simulink model "rigLoggerRigH"  (R2012b)
settings: Solver=FixedStepDiscrete  StartTime=0.0  StopTime=10.0  FixedStep=0.001  RelTol=1e-3
undefined symbols (not defined in the file or in its folder): macaddr
libraries: Lib_FileLogger x10, xpcnetworkbufferlib x1, xpcethernetlib x1
settings Model: BufferReuse=off  Creator=gilja  LastModifiedBy=Chethan
settings SolverCC: EnableConcurrentExecution=on  ConcurrentTasks=on
settings DataIOCC: SaveOutput=off  SignalLogging=off  SaveTime=off
settings OptimizationCC: InlineParams=on  InlineInvariantSignals=on  OptimizeBlockIOStorage=off  BufferReuse=off  ExpressionFolding=off  LocalBlockOutputs=off  SimCompilerOptimization=On
settings HardwareCC: ProdIntDivRoundTo=Zero  ProdEndianess=LittleEndian  ProdHWDeviceType=Generic->32-bit x86 compatible
settings ModelReferenceCC: ModelReferenceNumInstancesAllowed=Single  ModelReferenceMinAlgLoopOccurrences=on
settings RTWCC: SystemTargetFile=xpctarget.tlc  TemplateMakefile=xpc_default_tmf  Description=xPC Target  ProcessScript=xpctarget_make_rtw_hook  RTWCompilerOptimization=On
settings CodeAppCC: MaxIdLength=62
settings xpcTargetCC: TargetFcnLib=ansi_tfl_table_tmw.mat  CodeReplacementLibrary=XPC_BLAS  ParMdlRefBuildCompliant=on  ConcurrentExecutionCompliant=on  CombineSignalStateStructs=off  GRTInterface=on  RL32LogTETModifier=off  xPCTaskExecutionProfile=off  xPCRL32EventNumber=5000  xPCisDownloadable=off  xPCLoadParamSetFile=off  xPCConcurrentTasks=off  xPCEnableSFAnimation=off

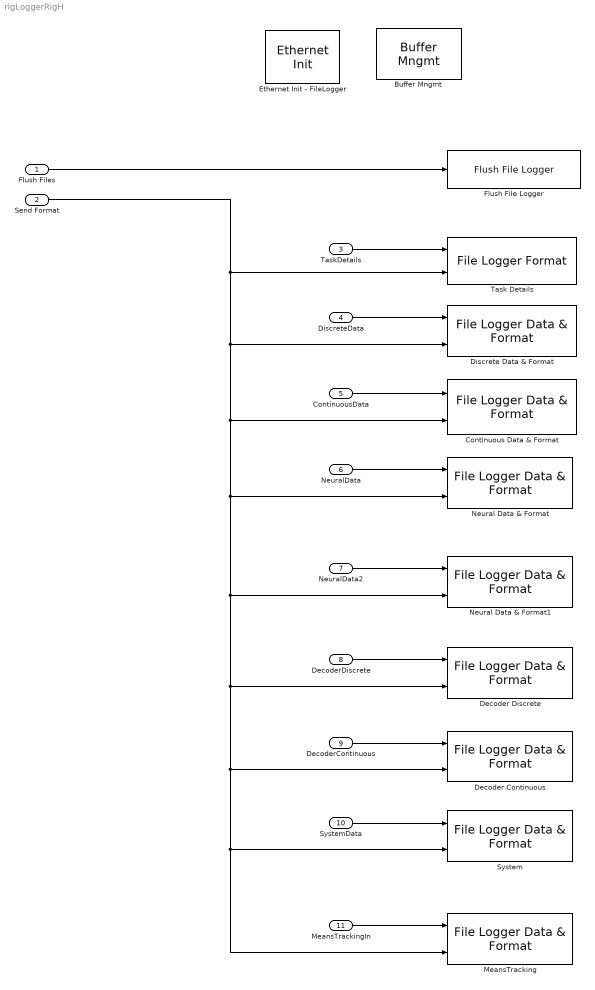
== system rigLoggerRigH ==
  Flush Files : Inport  OutDataTypeStr=boolean
  Send Format : Inport  Port=2  OutDataTypeStr=boolean
  TaskDetails : Inport  Port=3  OutDataTypeStr=Bus: fileLoggerFormat
  DiscreteData : Inport  Port=4  OutDataTypeStr=Bus: fileLoggerFormatAndData
  ContinuousData : Inport  Port=5  OutDataTypeStr=Bus: fileLoggerFormatAndData
  NeuralData : Inport  Port=6  OutDataTypeStr=Bus: fileLoggerFormatAndData
  NeuralData2 : Inport  Port=7  OutDataTypeStr=Bus: fileLoggerFormatAndData
  DecoderDiscrete : Inport  Port=8  OutDataTypeStr=Bus: fileLoggerFormatAndData
  DecoderContinuous : Inport  Port=9  OutDataTypeStr=Bus: fileLoggerFormatAndData
  SystemData : Inport  Port=10  OutDataTypeStr=Bus: fileLoggerFormatAndData
  MeansTrackingIn : Inport  Port=11  OutDataTypeStr=Bus: fileLoggerFormatAndData
  "Buffer Mngmt " : xpcnetworkbufferlib/Buffer Mngmt   Priority=-1  SampleTime=-1  PoolSizes=[8196 512 4096 65535]  ShowTune=on
  Continuous Data & Format : Lib_FileLogger/File Logger Data & Format
  Decoder Continuous : Lib_FileLogger/File Logger Data & Format
  Decoder Discrete : Lib_FileLogger/File Logger Data & Format
  Discrete Data & Format : Lib_FileLogger/File Logger Data & Format
  Ethernet Init - FileLogger : xpcethernetlib/Ethernet Init   Priority=-1  ID=2  Driver=Intel Gigabit  Bus=6  Slot=0  SampleTime=-1  AddressSource=Specify  MAC=macaddr('00:00:00:00:00:00')  TxSA=off  RxPromiscuous=off  Multicast={}  RxBad=off  RxShort=off  MaxMTU=1518  TxThreshold=10  TxBuffers=128  RxBuffers=8  ShowTune=on  NumRxBlks=1
  Flush File Logger : Lib_FileLogger/Flush File Logger
  MeansTracking : Lib_FileLogger/File Logger Data & Format
  Neural Data & Format : Lib_FileLogger/File Logger Data & Format
  Neural Data & Format1 : Lib_FileLogger/File Logger Data & Format
  System : Lib_FileLogger/File Logger Data & Format
  Task Details : Lib_FileLogger/File Logger Format
  wires:
  Flush Files/1 -> Flush File Logger/1
  TaskDetails/1 -> Task Details/1
  ContinuousData/1 -> Continuous Data & Format/1
  DiscreteData/1 -> Discrete Data & Format/1
  NeuralData/1 -> Neural Data & Format/1
  DecoderDiscrete/1 -> Decoder Discrete/1
  DecoderContinuous/1 -> Decoder Continuous/1
  Send Format/1 -> Neural Data & Format1/2, MeansTracking/2, System/2, Decoder Continuous/2, Decoder Discrete/2, Neural Data & Format/2, Continuous Data & Format/2, Discrete Data & Format/2, Task Details/2
  NeuralData2/1 -> Neural Data & Format1/1
  SystemData/1 -> System/1
  MeansTrackingIn/1 -> MeansTracking/1
